simulink model "raCBF_ClosedLoop"  (R2024b)
settings: Solver=ode45  StartTime=0.0  StopTime=60  RelTol=1e-6  AbsTol=1e-8
settings Model: Creator=LAPTOPASADI  LastModifiedBy=LAPTOPASADI

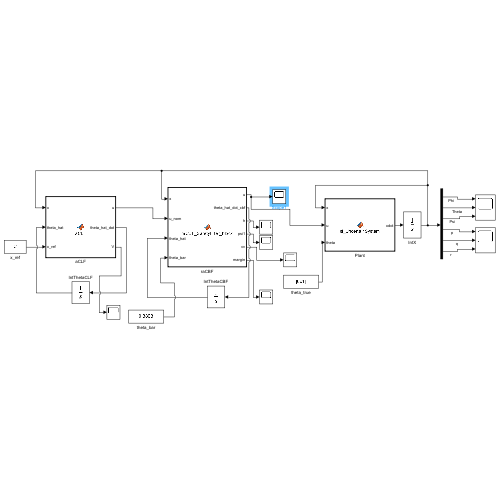
[thumbnail: Simulink's stored preview of the top-level diagram]
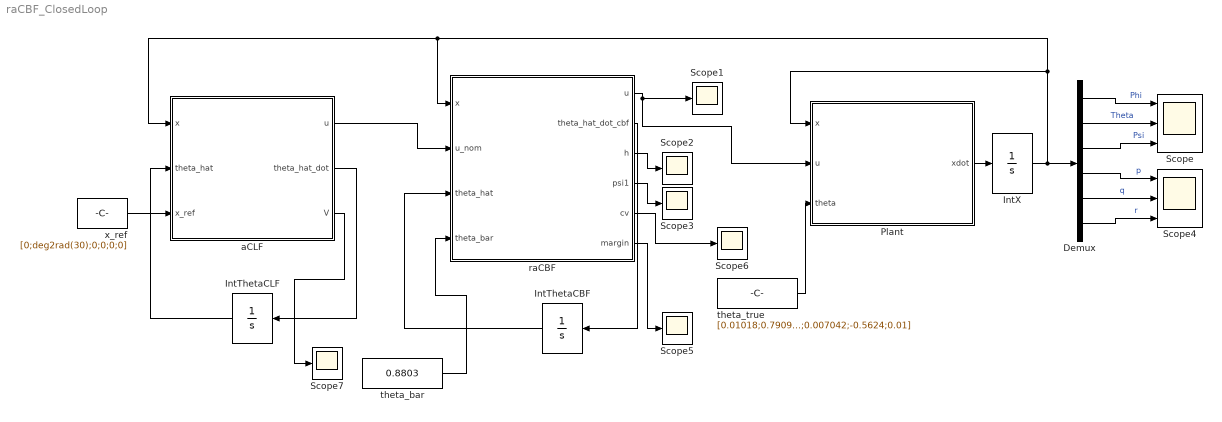
== system raCBF_ClosedLoop ==
  Demux : Demux  Outputs=6
  IntThetaCBF : Integrator  InitialCondition=[0;0.5;0.5;0;-0.3;0]
  IntThetaCLF : Integrator  InitialCondition=[0;0.5;0.5;0;-0.3;0]
  IntX : Integrator  InitialCondition=[-deg2rad(5);deg2rad(15);-deg2rad(20);0.2;-0.1;0.3]
  Plant : MATLAB Function  TreatAsAtomicUnit=on
  Scope : Scope  NumInputPorts=3
  Scope{1..3,5..7} (6 alike) : Scope
  Scope4 : Scope  NumInputPorts=3
  aCLF : MATLAB Function  TreatAsAtomicUnit=on
  raCBF : MATLAB Function  TreatAsAtomicUnit=on
  theta_bar : Constant  Value=0.8803
  theta_true : Constant  Value=[0.01018;0.7909;0.9366;0.007042;-0.5624;0.01]
  x_ref : Constant  Value=[0;deg2rad(30);0;0;0;0]
  wires:
  IntX/1 -> Demux/1, Plant/1(x), raCBF/1(x), aCLF/1(x)
  IntThetaCLF/1 -> aCLF/2(theta_hat)
  x_ref/1 -> aCLF/3(x_ref)
  aCLF/1(u) -> raCBF/2(u_nom)
  IntThetaCBF/1 -> raCBF/3(theta_hat)
  theta_bar/1 -> raCBF/4(theta_bar)
  aCLF/2(theta_hat_dot) -> IntThetaCLF/1
  raCBF/2(theta_hat_dot_cbf) -> IntThetaCBF/1
  raCBF/1(u) -> Scope1/1, Plant/2(u)
  theta_true/1 -> Plant/3(theta)
  Plant/1(xdot) -> IntX/1
  raCBF/3(h) -> Scope2/1
  raCBF/6(margin) -> Scope5/1
  Demux/4 -> Scope4/1  "p"
  Demux/1 -> Scope/1  "Phi"
  Demux/2 -> Scope/2  "Theta"
  Demux/5 -> Scope4/2  "q"
  Demux/6 -> Scope4/3  "r"
  Demux/3 -> Scope/3  "Psi"
  raCBF/4(psi1) -> Scope3/1
  raCBF/5(cv) -> Scope6/1
  aCLF/3(V) -> Scope7/1

== matlab function raCBF_ClosedLoop/aCLF ==
  data: x input; u output; theta_hat input; x_ref input; theta_hat_dot output; V output
function [u, theta_hat_dot, V] = aCLF(x, theta_hat, x_ref)
%#codegen
    coder.extrinsic('lyap','quadprog','optimoptions');

    gamma_clf = 0.5;
    Gamma     = 10*eye(6);
    u_min     = -0.1;  u_max = 0.1;

    Ixx = 0.0043;  Iyy = 0.0142;  Izz = 0.0176;  Ixz = 1e-4;
    dcg = 0.175;   hcg = 0.085;   d_over_b = 1.2e-6/3.13e-5;
    I = [ Ixx,0,-Ixz; 0,Iyy,0; -Ixz,0,Izz];
    B_alloc = [0,0,dcg,d_over_b;  0,hcg,0,0;  0,0,d_over_b,-dcg];
    Acl = [zeros(3),eye(3); -4*eye(3),-4*eye(3)];
    P = zeros(6);  P = lyap(Acl', 0.1*eye(6));

    phi = x(1);  th = x(2);
    p = x(4);  q = x(5);  r = x(6);
    omega = [p; q; r];

    y = [phi; th; x(3)] - x_ref(1:3);
    [J, dJdphi, dJdth] = euler_J(phi, th);
    y_dot = J*omega;

    eta = [y; y_dot];
    V   = eta'*P*eta;
    P11 = P(1:3,1:3); P12 = P(1:3,4:6); P22 = P(4:6,4:6);

    J_dot  = dJdphi*y_dot(1) + dJdth*y_dot(2);
    alpha0 = J_dot*omega;

    F_omega = [ p*q,-q*r,0,0,0,-p;  0,0,p*r,-(p^2-r^2),0,-q;  -q*r,0,0,0,p*q,-r];
    G_omega = I \ B_alloc;
    alpha_F = J * F_omega;
    A_dec   = J * G_omega;

    sigma     = 2*(y'*P12 + y_dot'*P22);
    omega_clf = 2*(y'*P11 + y_dot'*P12')*y_dot + sigma*alpha0;
    phi_clf   = alpha_F' * sigma';
    LgV       = sigma * A_dec;

    b_clf = -omega_clf - phi_clf'*theta_hat - gamma_clf*V;

    H    = 2*eye(4);
    f_qp = zeros(4,1);
    lb   = u_min*ones(4,1);
    ub   = u_max*ones(4,1);
    opts = optimoptions('quadprog','Display','off');

    u    = zeros(4,1);
    flag = 0;
    [u, ~, flag] = quadprog(H, f_qp, LgV, b_clf, [], [], lb, ub, [], opts);
    if flag < 0, u = zeros(4,1); end

    theta_hat_dot = Gamma * phi_clf;
end

function [J, dJdphi, dJdth] = euler_J(phi, th)
    cphi = cos(phi);  sphi = sin(phi);
    cth  = cos(th);   sth  = sin(th);
    if abs(cth) < 1e-6, cth = sign(cth + 1e-6)*1e-6; end
    tth = sth/cth;  sec2 = 1/cth^2;
    J      = [1, sphi*tth, cphi*tth;  0, cphi, -sphi;  0, sphi/cth, cphi/cth];
    dJdphi = [0, cphi*tth,-sphi*tth;  0,-sphi,-cphi;   0, cphi/cth,-sphi/cth];
    dJdth  = [0, sphi*sec2,    cphi*sec2;
              0, 0,            0;
              0, sphi*sth*sec2,cphi*sth*sec2];
end

== matlab function raCBF_ClosedLoop/Plant ==
  data: x input; u input; xdot output; theta input
function xdot = sl_UncertainSystem(x, u, theta)
%#codegen
% MATLAB Function block for  Uncertain_System.slx.
% Inputs : x (6), u (4), theta (6)
% Output : xdot (6) so that  xdot = f0(x) + F(x)*theta + g(x)*u.

    Ixx = 0.0043;  Iyy = 0.0142;  Izz = 0.0176;  Ixz = 1e-4;
    dcg = 0.175;   hcg = 0.085;   d_over_b = 1.2e-6 / 3.13e-5;

    I = [ Ixx, 0, -Ixz;  0, Iyy, 0;  -Ixz, 0, Izz];
    B_alloc = [0, 0,   dcg,        d_over_b;
               0, hcg, 0,          0;
               0, 0,   d_over_b,  -dcg];

    phi = x(1);  th = x(2);
    p   = x(4);  q  = x(5);  r = x(6);
    omega = [p; q; r];

    cphi = cos(phi);  sphi = sin(phi);
    cth  = cos(th);   sth  = sin(th);
    if abs(cth) < 1e-6, cth = sign(cth + 1e-6)*1e-6; end
    tth = sth/cth;

    J = [1, sphi*tth, cphi*tth;
         0, cphi,    -sphi;
         0, sphi/cth, cphi/cth];

    F_omega = [ p*q, -q*r, 0,    0,           0,   -p;
                0,    0,   p*r, -(p^2 - r^2), 0,   -q;
               -q*r,  0,   0,    0,           p*q, -r];

    f0    = [J*omega; 0; 0; 0];
    F_reg = [zeros(3,6); F_omega];
    g     = [zeros(3,4); I \ B_alloc];

    xdot = f0 + F_reg*theta + g*u;
end

== matlab function raCBF_ClosedLoop/raCBF ==
  data: x input; u output; u_nom input; theta_hat input; theta_bar input; theta_hat_dot_cbf output; h output; psi1 output; cv output; margin output
function [u, theta_hat_dot_cbf, h, psi1, cv, margin] = raCBF_SafetyFilter_block( ...
                                                  x, u_nom, theta_hat, theta_bar)
%#codegen
% Robust adaptive CBF safety filter for the Simulink MATLAB Function block.
% Same HOCBF as the aCBF version, but the constraint RHS is tightened by
%   ||phi_h(x)|| * theta_bar
% to guarantee  hdot >= -gamma_B*h  for every admissible parameter error.
%
% Inputs : x (6), u_nom (4), theta_hat (6), theta_bar (1)
% Outputs: u (4), theta_hat_dot_cbf (6), h, psi1, cv, margin

    coder.extrinsic('quadprog','optimoptions');

    % ---------- constants ----------
    theta_max = deg2rad(20);
    alpha1    = 5;
    alpha2    = 5;
    Gamma     = 10*eye(6);
    u_min     = -0.1;  u_max = 0.1;

    Ixx = 0.0043;  Iyy = 0.0142;  Izz = 0.0176;  Ixz = 1e-4;
    dcg = 0.175;   hcg = 0.085;   d_over_b = 1.2e-6/3.13e-5;
    I = [ Ixx,0,-Ixz; 0,Iyy,0; -Ixz,0,Izz];
    B_alloc = [0,0,dcg,d_over_b;  0,hcg,0,0;  0,0,d_over_b,-dcg];
    G_omega = I \ B_alloc;

    % ---------- state extraction ----------
    phi = x(1);  th = x(2);
    p   = x(4);  q  = x(5);  r = x(6);
    omega = [p; q; r];

    cphi = cos(phi);  sphi = sin(phi);
    cth  = cos(th);   sth  = sin(th);
    if abs(cth) < 1e-6, cth = sign(cth + 1e-6)*1e-6; end

    % ---------- HOCBF chain ----------
    h         = theta_max - th;
    J2        = [0, cphi, -sphi];
    theta_dot = J2 * omega;
    h_dot     = -theta_dot;
    psi1      = h_dot + alpha1 * h;

    phi_dot      = p + sphi*(sth/cth)*q + cphi*(sth/cth)*r;
    J2_dot_omega = -sphi*phi_dot*q - cphi*phi_dot*r;

    F_omega = [ p*q,-q*r,0,0,0,-p;
                0,0,p*r,-(p^2 - r^2),0,-q;
               -q*r,0,0,0,p*q,-r];

    Lf_psi1 = -J2_dot_omega - alpha1 * theta_dot;
    phi_h   = -(J2 * F_omega)';
    Lg_psi1 = -(J2 * G_omega);

    % ---------- robustness margin ----------
    margin = norm(phi_h) * theta_bar;

    % ---------- safety-filter QP (tightened by margin) ----------
    H    = 2*eye(4);
    f_qp = -2*u_nom;
    A    = -Lg_psi1;
    b    = Lf_psi1 + phi_h'*theta_hat + alpha2*psi1 - margin;
    lb   = u_min*ones(4,1);
    ub   = u_max*ones(4,1);
    opts = optimoptions('quadprog','Display','off');

    % Default = saturated u_nom; overwrite only on solver success.
    u = min(max(u_nom, u_min), u_max);

    [uRaw, ~, flagRaw] = quadprog(H, f_qp, A, b, [], [], lb, ub, u_nom, opts);
    flag = -1;  flag = double(flagRaw);
    if flag > 0
        for k = 1:4
            u(k) = double(uRaw(k));
        end
        u = min(max(u, u_min), u_max);
    end

    % ---------- constraint value (for scoping) ----------
    cv = Lf_psi1 + phi_h'*theta_hat + Lg_psi1*u + alpha2*psi1 - margin;

    % ---------- CBF-side parameter update law ----------
    theta_hat_dot_cbf = -Gamma * phi_h;
end
